simulink model "sim1"  (R2024a)
settings: Solver=FixedStepAuto  StartTime=0.0  StopTime=10.0  FixedStep=1  RelTol=1e-3
settings Model: Creator=alexe  LastModifiedBy=alexe

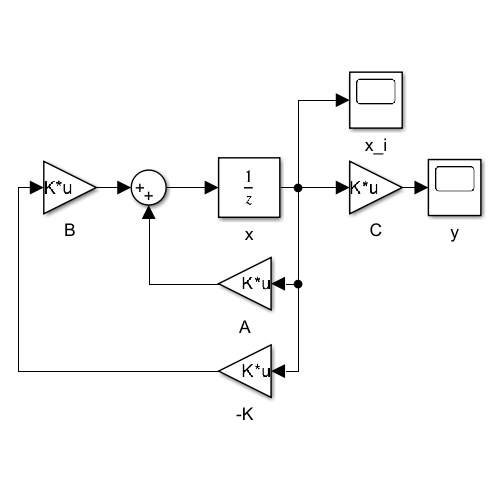
[thumbnail: Simulink's stored preview of the top-level diagram]
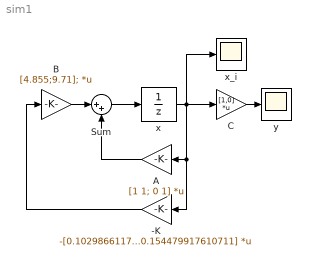
== system sim1 ==
  -K : Gain  Gain=-[0.102986611740474,0.154479917610711]  Multiplication=Matrix(K*u)
  A : Gain  Gain=[1 1; 0 1]  Multiplication=Matrix(K*u)
  B : Gain  Gain=[4.855;9.71];  Multiplication=Matrix(K*u)
  C : Gain  Gain=[1,0]  Multiplication=Matrix(K*u)
  Sum : Sum  Inputs=|++
  x : UnitDelay  InitialCondition=[1;0];  SampleTime=-1  HasFrameUpgradeWarning=on
  x_i : Scope
  y : Scope
  wires:
  Sum/1 -> x/1
  x/1 -> x_i/1, C/1, -K/1, A/1
  A/1 -> Sum/2
  B/1 -> Sum/1
  -K/1 -> B/1
  C/1 -> y/1
